simulink model "Full_TRC"  (R2014a)
settings: Solver=ode45  StartTime=0.0  StopTime=10.0  RelTol=1e-3
values from neighbouring files (symbols this model uses):
  Beta = 0    [Full_TRC_val.m]
settings Model: Creator=Nathan  LastModifiedBy=Nathan
settings DebuggingCC: UnderspecifiedInitializationDetection=Classic  StateNameClashWarn=warning

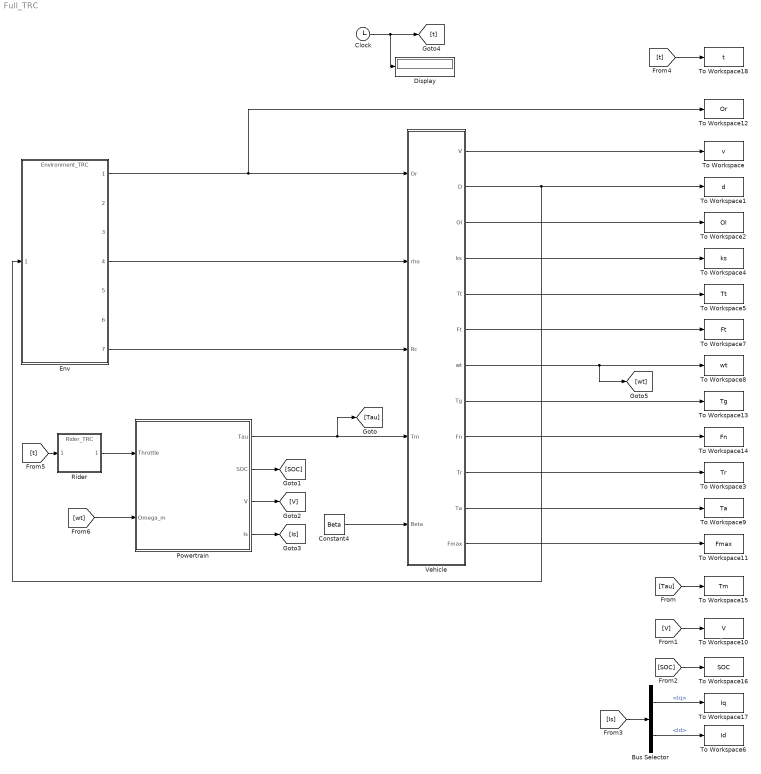
== system Full_TRC ==
  Bus Selector : BusSelector  OutputSignals=Iq,Id
  Clock : Clock
  Constant4 : Constant  Value=Beta
  Display : Display
  Env : ModelReference  ModelNameDialog=Environment_TRC.slx  SimulationMode=Normal  ModelReferenceVersion=1.17  CopyOfModelName=Environment_TRC.slx  DefaultDataLogging=on
  Powertrain : Subsystem
  Rider : ModelReference  ModelNameDialog=Rider_TRC.slx  SimulationMode=Normal  ModelReferenceVersion=1.3  CopyOfModelName=Rider_TRC.slx  DefaultDataLogging=on
  To Workspace : ToWorkspace  VariableName=v  SampleTime=-1
  To Workspace1 : ToWorkspace  VariableName=d  SampleTime=-1
  To Workspace10 : ToWorkspace  VariableName=V  SampleTime=-1
  To Workspace11 : ToWorkspace  VariableName=Fmax  SampleTime=-1
  To Workspace12 : ToWorkspace  VariableName=Or  SampleTime=-1
  To Workspace13 : ToWorkspace  VariableName=Tg  SampleTime=-1
  To Workspace14 : ToWorkspace  VariableName=Fn  SampleTime=-1
  To Workspace15 : ToWorkspace  VariableName=Tm  SampleTime=-1
  To Workspace16 : ToWorkspace  VariableName=SOC  SampleTime=-1
  To Workspace17 : ToWorkspace  VariableName=Iq  SampleTime=-1
  To Workspace18 : ToWorkspace  VariableName=t  SampleTime=-1
  To Workspace2 : ToWorkspace  VariableName=Ol  SampleTime=-1
  To Workspace3 : ToWorkspace  VariableName=Tr  SampleTime=-1
  To Workspace4 : ToWorkspace  VariableName=ks  SampleTime=-1
  To Workspace5 : ToWorkspace  VariableName=Tt  SampleTime=-1
  To Workspace6 : ToWorkspace  VariableName=Id  SampleTime=-1
  To Workspace7 : ToWorkspace  VariableName=Ft  SampleTime=-1
  To Workspace8 : ToWorkspace  VariableName=wt  SampleTime=-1
  To Workspace9 : ToWorkspace  VariableName=Ta  SampleTime=-1
  Vehicle : Subsystem
  wires:
  Clock/1 -> [t], Display/1
  Constant4/1 -> Vehicle/5(Beta)
  Vehicle/6(Ft) -> To Workspace7/1
  Vehicle/1(V) -> To Workspace/1
  Vehicle/2(D) -> Env/1, To Workspace1/1
  Vehicle/3(Ol) -> To Workspace2/1
  Vehicle/4(ks) -> To Workspace4/1
  Vehicle/5(Tt) -> To Workspace5/1
  Vehicle/7(wt) -> [wt], To Workspace8/1
  Vehicle/8(Tg) -> To Workspace13/1
  Vehicle/9(Fn) -> To Workspace14/1
  Vehicle/10(Tr) -> To Workspace3/1
  Vehicle/11(Ta) -> To Workspace9/1
  Vehicle/12("Fmax ") -> To Workspace11/1
  Powertrain/1(Tau) -> [Tau], Vehicle/4(Tm)
  Env/1 -> To Workspace12/1, Vehicle/1(Or)
  Env/4 -> Vehicle/2(rho)
  Env/7 -> Vehicle/3(Rc)
  [Tau] -> To Workspace15/1
  Powertrain/2(SOC) -> [SOC]
  Powertrain/3(V) -> [V]
  Powertrain/4(Is) -> [Is]
  [V] -> To Workspace10/1
  [SOC] -> To Workspace16/1
  Rider/1 -> Powertrain/1(Throttle)
  [t] -> To Workspace18/1
  [t] -> Rider/1
  [wt] -> Powertrain/2(Omega_m)
  [Is] -> Bus Selector/1
  Bus Selector/1 -> To Workspace17/1  "<Iq>"
  Bus Selector/2 -> To Workspace6/1  "<Id>"

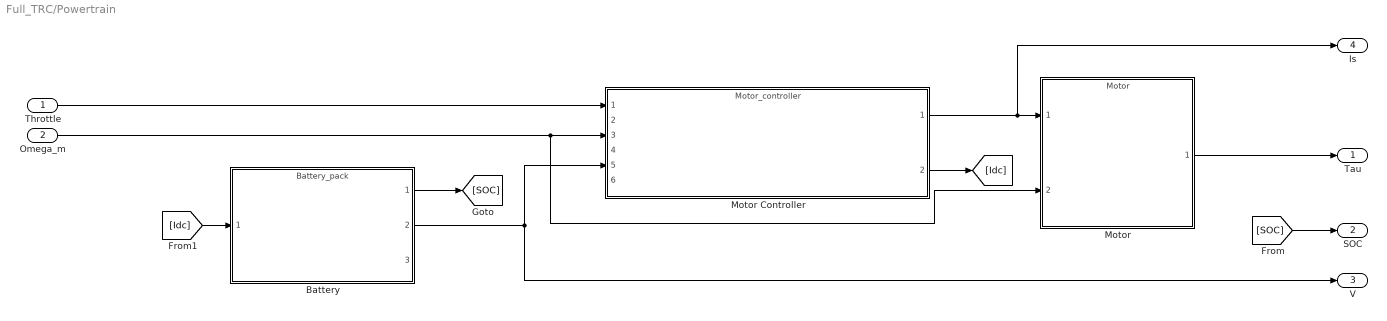
== system Full_TRC/Powertrain ==
  Throttle : Inport
  Omega_m : Inport  Port=2
  Battery : ModelReference  ModelNameDialog=Battery_pack.slx  SimulationMode=Normal  ModelReferenceVersion=1.27  CopyOfModelName=Battery_pack.slx  DefaultDataLogging=on
  Motor : ModelReference  ModelNameDialog=Motor.slx  SimulationMode=Normal  ModelReferenceVersion=1.41  CopyOfModelName=Motor.slx  DefaultDataLogging=on
  Motor Controller : ModelReference  ModelNameDialog=Motor_controller.slx  SimulationMode=Normal  ModelReferenceVersion=1.14  CopyOfModelName=Motor_controller.slx  DefaultDataLogging=on
  Tau : Outport
  SOC : Outport  Port=2
  V : Outport  Port=3
  Is : Outport  Port=4
  wires:
  Motor Controller/1 -> Is/1, Motor/1
  Omega_m/1 -> Motor/2, Motor Controller/3
  Throttle/1 -> Motor Controller/1
  Battery/2 -> V/1, Motor Controller/5
  Motor/1 -> Tau/1
  Battery/1 -> [SOC]
  [SOC] -> SOC/1
  Motor Controller/2 -> [Idc]
  [Idc] -> Battery/1

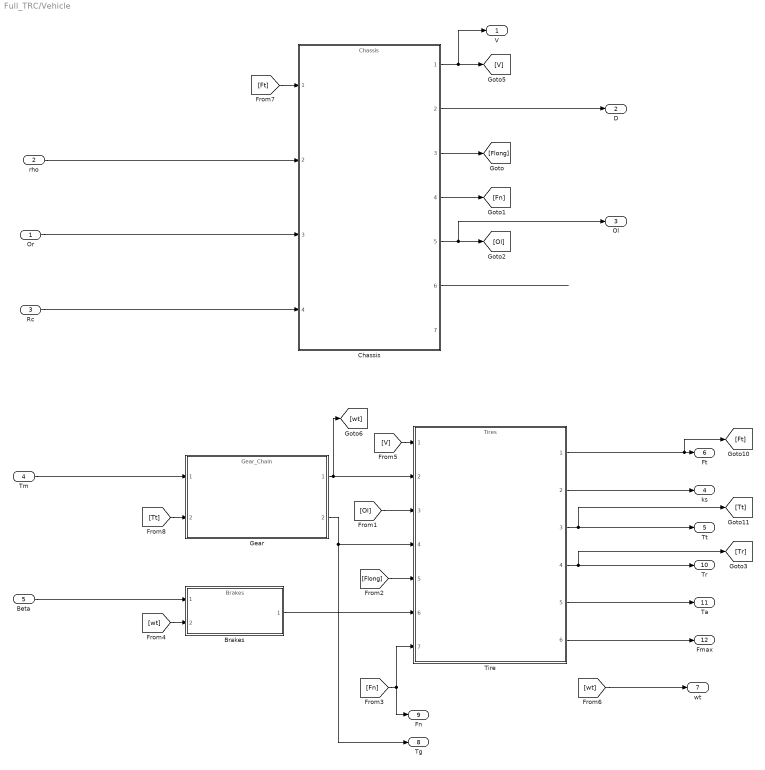
== system Full_TRC/Vehicle ==
  Or : Inport
  rho : Inport  Port=2
  Rc : Inport  Port=3
  Tm : Inport  Port=4
  Beta : Inport  Port=5
  Brakes : ModelReference  ModelNameDialog=Brakes.slx  SimulationMode=Normal  ModelReferenceVersion=1.7  CopyOfModelName=Brakes.slx  DefaultDataLogging=on
  Chassis : ModelReference  ModelNameDialog=Chassis.slx  SimulationMode=Normal  ModelReferenceVersion=1.18  CopyOfModelName=Chassis.slx  DefaultDataLogging=on
  Gear : ModelReference  ModelNameDialog=Gear_Chain.slx  SimulationMode=Normal  ModelReferenceVersion=1.17  CopyOfModelName=Gear_Chain.slx  DefaultDataLogging=on
  Tire : ModelReference  ModelNameDialog=Tires.slx  SimulationMode=Normal  ModelReferenceVersion=1.79  CopyOfModelName=Tires.slx  DefaultDataLogging=on
  V : Outport
  D : Outport  Port=2
  Ol : Outport  Port=3
  ks : Outport  Port=4
  Tt : Outport  Port=5
  Ft : Outport  Port=6
  wt : Outport  Port=7
  Tg : Outport  Port=8
  Fn : Outport  Port=9
  Tr : Outport  Port=10
  Ta : Outport  Port=11
  "Fmax " : Outport  Port=12
  wires:
  Chassis/3 -> [Flong]
  [Ol] -> Tire/3
  Chassis/4 -> [Fn]
  Chassis/5 -> Ol/1, [Ol]
  Gear/1 -> Tire/2, [wt]
  [Tt] -> Gear/2
  [Ft] -> Chassis/1
  Gear/2 -> Tg/1, Tire/4
  [wt] -> Brakes/2
  [V] -> Tire/1
  [Fn] -> Tire/7, Fn/1
  Chassis/1 -> V/1, [V]
  [Flong] -> Tire/5
  Chassis/6 -> ?
  Or/1 -> Chassis/3
  Beta/1 -> Brakes/1
  Tm/1 -> Gear/1
  Rc/1 -> Chassis/4
  rho/1 -> Chassis/2
  Tire/1 -> Ft/1, [Ft]
  [wt] -> wt/1
  Brakes/1 -> Tire/6
  Chassis/2 -> D/1
  Tire/2 -> ks/1
  Tire/3 -> [Tt], Tt/1
  Tire/4 -> [Tr], Tr/1
  Tire/5 -> Ta/1
  Tire/6 -> "Fmax "/1
